simulink library "corr_3ghz_10_1_lib"  (Simulink 7.0)
libraries: xbsIndex_r4 x29, corr_3ghz_10_1_lib x6, casper_library x6
settings Model: Creator=wjm  LastModifiedBy=wjm

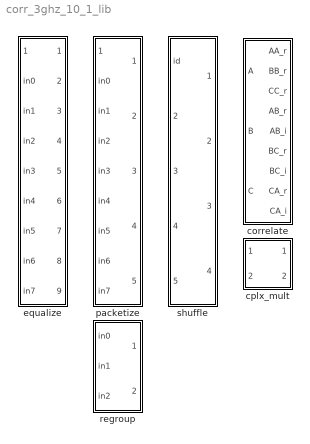
== system corr_3ghz_10_1_lib ==
  correlate : Subsystem
  cplx_mult : Subsystem
  equalize : Subsystem
  packetize : Subsystem
  regroup : Subsystem
  shuffle : Subsystem

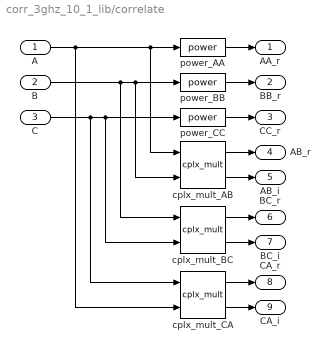
== system corr_3ghz_10_1_lib/correlate ==
  A : Inport  OutDataType=sfix(16)  OutScaling=2^0
  B : Inport  Port=2  OutDataType=sfix(16)  OutScaling=2^0
  C : Inport  Port=3  OutDataType=sfix(16)  OutScaling=2^0
  cplx_mult_AB : corr_3ghz_10_1_lib/cplx_mult  SystemSampleTime=-1
  cplx_mult_BC : corr_3ghz_10_1_lib/cplx_mult  SystemSampleTime=-1
  cplx_mult_CA : corr_3ghz_10_1_lib/cplx_mult  SystemSampleTime=-1
  power_AA : casper_library/Misc/power  SystemSampleTime=-1  BitWidth=8
  power_BB : casper_library/Misc/power  SystemSampleTime=-1  BitWidth=8
  power_CC : casper_library/Misc/power  SystemSampleTime=-1  BitWidth=8
  AA_r : Outport  OutDataType=sfix(16)  OutScaling=2^0
  BB_r : Outport  Port=2  OutDataType=sfix(16)  OutScaling=2^0
  CC_r : Outport  Port=3  OutDataType=sfix(16)  OutScaling=2^0
  AB_r : Outport  Port=4  OutDataType=sfix(16)  OutScaling=2^0
  AB_i : Outport  Port=5  OutDataType=sfix(16)  OutScaling=2^0
  BC_r : Outport  Port=6  OutDataType=sfix(16)  OutScaling=2^0
  BC_i : Outport  Port=7  OutDataType=sfix(16)  OutScaling=2^0
  CA_r : Outport  Port=8  OutDataType=sfix(16)  OutScaling=2^0
  CA_i : Outport  Port=9  OutDataType=sfix(16)  OutScaling=2^0
  wires:
  cplx_mult_BC/1 -> BC_r/1
  cplx_mult_AB/2 -> AB_i/1
  cplx_mult_AB/1 -> AB_r/1
  power_CC/1 -> CC_r/1
  power_BB/1 -> BB_r/1
  power_AA/1 -> AA_r/1
  A/1 -> cplx_mult_AB/1, power_AA/1, cplx_mult_CA/2
  B/1 -> cplx_mult_AB/2, power_BB/1, cplx_mult_BC/1
  C/1 -> cplx_mult_BC/2, power_CC/1, cplx_mult_CA/1
  cplx_mult_CA/2 -> CA_i/1
  cplx_mult_CA/1 -> CA_r/1
  cplx_mult_BC/2 -> BC_i/1

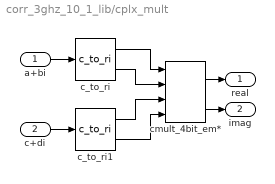
== system corr_3ghz_10_1_lib/cplx_mult ==
  a+bi : Inport  OutDataType=sfix(16)  OutScaling=2^0
  c+di : Inport  Port=2  OutDataType=sfix(16)  OutScaling=2^0
  c_to_ri : casper_library/Misc/c_to_ri  SystemSampleTime=-1  n_bits=8  bin_pt=7
      settings: AttributesFormatString=8_7 r/i
  c_to_ri1 : casper_library/Misc/c_to_ri  SystemSampleTime=-1  n_bits=8  bin_pt=7
      settings: AttributesFormatString=8_7 r/i
  cmult_4bit_em* : casper_library/Multipliers/cmult_4bit_em*  SystemSampleTime=-1  mult_latency=1  add_latency=0
  real : Outport  OutDataType=sfix(16)  OutScaling=2^0
  imag : Outport  Port=2  OutDataType=sfix(16)  OutScaling=2^0
  wires:
  cmult_4bit_em*/2 -> imag/1
  cmult_4bit_em*/1 -> real/1
  a+bi/1 -> c_to_ri/1
  c_to_ri/1 -> cmult_4bit_em*/1
  c+di/1 -> c_to_ri1/1
  c_to_ri1/2 -> cmult_4bit_em*/4
  c_to_ri/2 -> cmult_4bit_em*/2
  c_to_ri1/1 -> cmult_4bit_em*/3

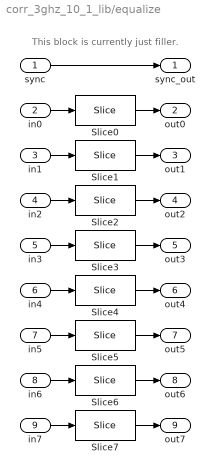
== system corr_3ghz_10_1_lib/equalize ==
  note: This block is currently just filler.
  sync : Inport
  in0 : Inport  Port=2
  in1 : Inport  Port=3
  in2 : Inport  Port=4
  in3 : Inport  Port=5
  in4 : Inport  Port=6
  in5 : Inport  Port=7
  in6 : Inport  Port=8
  in7 : Inport  Port=9
  Slice{0..7} (8 alike) : xbsIndex_r4/Slice  nbits=8  boolean_output=off  mode=Upper Bit Location + Width  bit1=0  base1=MSB of Input  bit0=0  base0=LSB of Input  dbl_ovrd=off  block_type=slice
      settings: infoedit="Extracts a given range of bits from each input sample and presents it at the output.  The output type is ordinarily unsigned with binary point at zero, but can be Boolean when the slice is one bit wide.<P><P>Hardware notes: In hardware this block costs nothing."  block_version=10.1.1
  sync_out : Outport
  out0 : Outport  Port=2
  out1 : Outport  Port=3
  out2 : Outport  Port=4
  out3 : Outport  Port=5
  out4 : Outport  Port=6
  out5 : Outport  Port=7
  out6 : Outport  Port=8
  out7 : Outport  Port=9
  wires:
  in0/1 -> Slice0/1
  Slice0/1 -> out0/1
  in1/1 -> Slice1/1
  in2/1 -> Slice2/1
  in3/1 -> Slice3/1
  Slice1/1 -> out1/1
  Slice2/1 -> out2/1
  Slice3/1 -> out3/1
  in4/1 -> Slice4/1
  Slice4/1 -> out4/1
  in5/1 -> Slice5/1
  in6/1 -> Slice6/1
  in7/1 -> Slice7/1
  Slice5/1 -> out5/1
  Slice6/1 -> out6/1
  Slice7/1 -> out7/1
  sync/1 -> sync_out/1

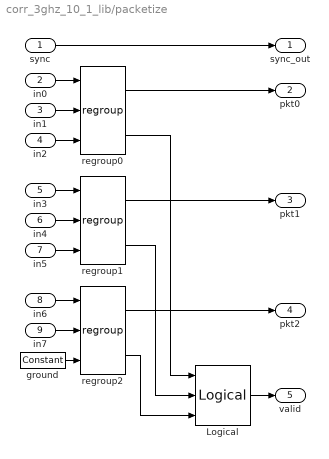
== system corr_3ghz_10_1_lib/packetize ==
  sync : Inport
  in0 : Inport  Port=2
  in1 : Inport  Port=3
  in2 : Inport  Port=4
  in3 : Inport  Port=5
  in4 : Inport  Port=6
  in5 : Inport  Port=7
  in6 : Inport  Port=8
  in7 : Inport  Port=9
  Logical : xbsIndex_r4/Logical  logical_function=AND  inputs=3  en=off  latency=0  precision=Full  arith_type=Unsigned  n_bits=16  bin_pt=0  align_bp=on  dbl_ovrd=off  block_type=logical
      settings: block_version=10.1.1
  ground : xbsIndex_r4/Constant  arith_type=Unsigned  const=0  n_bits=8  bin_pt=0  explicit_period=on  period=1  equ=P=C  opselect=C  inp2=PCIN>>17  opr=+  inp1=P  carry=CIN  dbl_ovrd=off  block_type=constant
      settings: block_version=10.1.1
  regroup0 : corr_3ghz_10_1_lib/regroup  SystemSampleTime=-1
  regroup1 : corr_3ghz_10_1_lib/regroup  SystemSampleTime=-1
  regroup2 : corr_3ghz_10_1_lib/regroup  SystemSampleTime=-1
  sync_out : Outport
  pkt0 : Outport  Port=2
  pkt1 : Outport  Port=3
  pkt2 : Outport  Port=4
  valid : Outport  Port=5
  wires:
  ground/1 -> regroup2/3
  in7/1 -> regroup2/2
  in6/1 -> regroup2/1
  in5/1 -> regroup1/3
  in4/1 -> regroup1/2
  in3/1 -> regroup1/1
  in2/1 -> regroup0/3
  in1/1 -> regroup0/2
  in0/1 -> regroup0/1
  regroup0/1 -> pkt0/1
  regroup1/1 -> pkt1/1
  regroup2/1 -> pkt2/1
  Logical/1 -> valid/1
  regroup0/2 -> Logical/1
  regroup1/2 -> Logical/2
  regroup2/2 -> Logical/3
  sync/1 -> sync_out/1

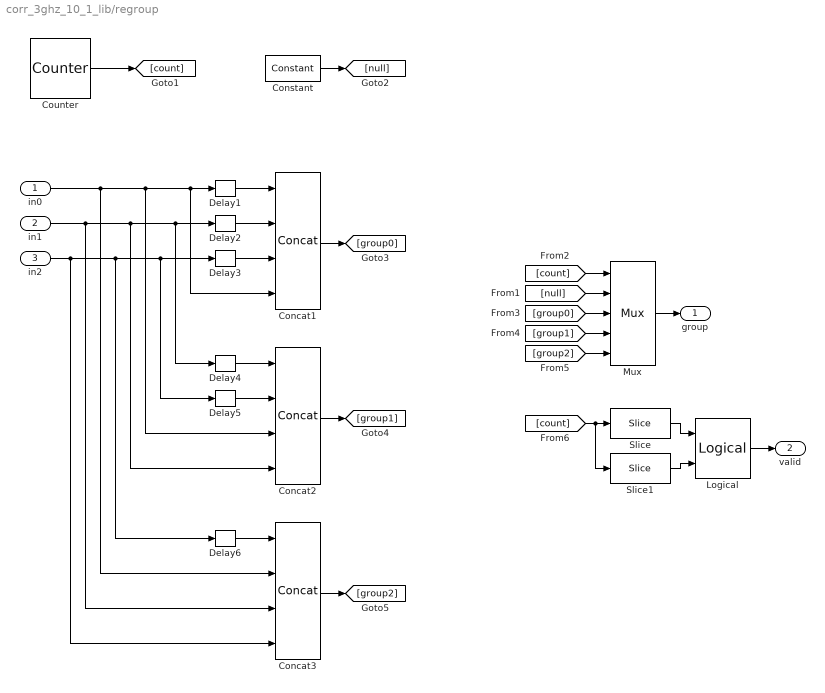
== system corr_3ghz_10_1_lib/regroup ==
  in0 : Inport  OutDataType=sfix(16)  OutScaling=2^0
  in1 : Inport  Port=2  OutDataType=sfix(16)  OutScaling=2^0
  in2 : Inport  Port=3  OutDataType=sfix(16)  OutScaling=2^0
  Concat1 : xbsIndex_r4/Concat  num_inputs=4  dbl_ovrd=off  block_type=concat
      settings: block_version=10.1.1
  Concat2 : xbsIndex_r4/Concat  num_inputs=4  dbl_ovrd=off  block_type=concat
      settings: block_version=10.1.1
  Concat3 : xbsIndex_r4/Concat  num_inputs=4  dbl_ovrd=off  block_type=concat
      settings: block_version=10.1.1
  Constant : xbsIndex_r4/Constant  arith_type=Unsigned  const=0  n_bits=32  bin_pt=0  explicit_period=on  period=1  equ=P=C  opselect=C  inp2=PCIN>>17  opr=+  inp1=P  carry=CIN  dbl_ovrd=off  block_type=constant
      settings: block_version=10.1.1
  Counter : xbsIndex_r4/Counter  cnt_type=Free Running  cnt_to=Inf  operation=Up  start_count=0  cnt_by_val=1  arith_type=Unsigned  n_bits=2  bin_pt=0  load_pin=off  rst=off  en=off  explicit_period=on  period=1  dbl_ovrd=off  use_behavioral_HDL=off  use_rpm=off  block_type=counter
      settings: block_version=10.1.1
  Delay{1..6} (6 alike) : xbsIndex_r4/Delay  en=off  latency=1  dbl_ovrd=off  reg_retiming=off  block_type=delay
      settings: block_version=10.1.1
  Logical : xbsIndex_r4/Logical  logical_function=OR  inputs=2  en=off  latency=0  precision=Full  arith_type=Unsigned  n_bits=16  bin_pt=0  align_bp=on  dbl_ovrd=off  block_type=logical
      settings: block_version=10.1.1
  Mux : xbsIndex_r4/Mux  inputs=4  en=off  latency=0  precision=User Defined  arith_type=Unsigned  n_bits=32  bin_pt=0  quantization=Truncate  overflow=Wrap  dbl_ovrd=off  block_type=mux
      settings: block_version=10.1.1
  Slice : xbsIndex_r4/Slice  nbits=1  boolean_output=on  mode=Upper Bit Location + Width  bit1=0  base1=MSB of Input  bit0=0  base0=LSB of Input  dbl_ovrd=off  block_type=slice
      settings: infoedit="Extracts a given range of bits from each input sample and presents it at the output.  The output type is ordinarily unsigned with binary point at zero, but can be Boolean when the slice is one bit wide.<P><P>Hardware notes: In hardware this block costs nothing."  block_version=10.1.1
  Slice1 : xbsIndex_r4/Slice  nbits=1  boolean_output=on  mode=Lower Bit Location + Width  bit1=0  base1=MSB of Input  bit0=0  base0=LSB of Input  dbl_ovrd=off  block_type=slice
      settings: infoedit="Extracts a given range of bits from each input sample and presents it at the output.  The output type is ordinarily unsigned with binary point at zero, but can be Boolean when the slice is one bit wide.<P><P>Hardware notes: In hardware this block costs nothing."  block_version=10.1.1
  group : Outport  OutDataType=sfix(16)  OutScaling=2^0
  valid : Outport  Port=2  OutDataType=sfix(16)  OutScaling=2^0
  wires:
  Delay1/1 -> Concat1/1
  Delay2/1 -> Concat1/2
  Delay3/1 -> Concat1/3
  Delay4/1 -> Concat2/1
  Delay5/1 -> Concat2/2
  Delay6/1 -> Concat3/1
  in0/1 -> Delay1/1, Concat1/4, Concat2/3, Concat3/2
  in1/1 -> Delay2/1, Delay4/1, Concat2/4, Concat3/3
  in2/1 -> Delay3/1, Delay5/1, Delay6/1, Concat3/4
  Counter/1 -> [count]
  Concat1/1 -> [group0]
  Concat2/1 -> [group1]
  Concat3/1 -> [group2]
  Constant/1 -> [null]
  [count] -> Mux/1
  [null] -> Mux/2
  [group0] -> Mux/3
  [group1] -> Mux/4
  [group2] -> Mux/5
  Mux/1 -> group/1
  [count] -> Slice/1, Slice1/1
  Slice/1 -> Logical/1
  Slice1/1 -> Logical/2
  Logical/1 -> valid/1

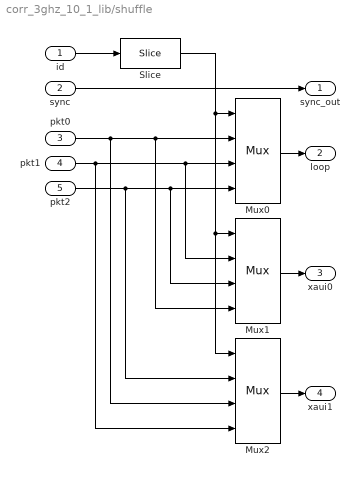
== system corr_3ghz_10_1_lib/shuffle ==
  id : Inport
  sync : Inport  Port=2
  pkt0 : Inport  Port=3
  pkt1 : Inport  Port=4
  pkt2 : Inport  Port=5
  Mux0 : xbsIndex_r4/Mux  inputs=3  en=off  latency=0  precision=Full  arith_type=Unsigned  n_bits=16  bin_pt=14  quantization=Truncate  overflow=Wrap  dbl_ovrd=off  block_type=mux
  Mux1 : xbsIndex_r4/Mux  inputs=3  en=off  latency=0  precision=Full  arith_type=Unsigned  n_bits=16  bin_pt=14  quantization=Truncate  overflow=Wrap  dbl_ovrd=off  block_type=mux
  Mux2 : xbsIndex_r4/Mux  inputs=3  en=off  latency=0  precision=Full  arith_type=Unsigned  n_bits=16  bin_pt=14  quantization=Truncate  overflow=Wrap  dbl_ovrd=off  block_type=mux
  Slice : xbsIndex_r4/Slice  nbits=2  boolean_output=off  mode=Upper Bit Location + Width  bit1=0  base1=MSB of Input  bit0=0  base0=LSB of Input  dbl_ovrd=off  block_type=slice
      settings: infoedit="Extracts a given range of bits from each input sample and presents it at the output.  The output type is ordinarily unsigned with binary point at zero, but can be Boolean when the slice is one bit wide.<P><P>Hardware notes: In hardware this block costs nothing."  block_version=10.1.1
  sync_out : Outport
  loop : Outport  Port=2
  xaui0 : Outport  Port=3
  xaui1 : Outport  Port=4
  wires:
  id/1 -> Slice/1
  pkt0/1 -> Mux0/2, Mux1/4, Mux2/3
  Mux0/1 -> loop/1
  pkt1/1 -> Mux0/3, Mux1/2, Mux2/4
  pkt2/1 -> Mux0/4, Mux1/3, Mux2/2
  Mux1/1 -> xaui0/1
  Mux2/1 -> xaui1/1
  sync/1 -> sync_out/1
  Slice/1 -> Mux1/1, Mux2/1, Mux0/1
